simulink model "torpedo_tom_ole__09_12_19_modell"  (R2019a)
settings: Solver=ode1  StartTime=0.0  StopTime=30  FixedStep=1e-4  RelTol=1e-3
values from neighbouring files (symbols this model uses):
  K_MESS = 1.0    (= 1)    [Hausaufgabe_Schiffeversenken_zum_16_12_19_Teil1.m]    (also in Hausaufgabe_Schiffeversenken_zum_16_12_19_Teil2.m; torpedo_tom_ole__09_12_19.m; torpedo_tom_ole__25_11_19.m)
  K_r = place(ss_A_Strecke,ss_B_Strecke,Placed_Poles)    [Hausaufgabe_Schiffeversenken_zum_16_12_19_Teil2.m]    (also in torpedo_tom_ole__09_12_19.m = place(ss_A,ss_B,Placed_Poles))
  P_VORFILTER = -(ss_C_Strecke*((ss_A_Strecke-ss_B_Strecke*K_r)^-1)*ss_B_Strecke)^-1    [Hausaufgabe_Schiffeversenken_zum_16_12_19_Teil2.m]    (also in torpedo_tom_ole__09_12_19.m = -(ss_C*((ss_A-ss_B*K_r)^-1)*ss_B)^-1)
  ss_A = [0 1 0 0; 0 0 a23 0; 0 0 0 1; 0 0 a43 0]    [V2_A4_ZR_separ_nonlin_Aufgabenstellung.m]    (also in rocket_task_definition.m; torpedo_tom_ole__09_12_19.m = [-1/T_RM 0 0; K_IS/T_NOMOTO -1/T_NOMOTO 0; 0 1 0])
  ss_B = [0; b2; 0; b4]    [V2_A4_ZR_separ_nonlin_Aufgabenstellung.m]    (also in rocket_task_definition.m; torpedo_tom_ole__09_12_19.m = [K_RM/T_RM; 0; 0])
  ss_C = [1 0 0 0; 0 1 0 0; 0 0 1 0; 0 0 0 1]    [V2_A4_ZR_separ_nonlin_Aufgabenstellung.m]    (also in rocket_task_definition.m; torpedo_tom_ole__09_12_19.m = [0 0 1])
  ss_D = zeros(n,1)    [V2_A4_ZR_separ_nonlin_Aufgabenstellung.m]    (also in rocket_task_definition.m; torpedo_tom_ole__09_12_19.m = 0)
  T_MESS = 0.5    [Hausaufgabe_Schiffeversenken_zum_16_12_19_Teil1.m]    (also in Hausaufgabe_Schiffeversenken_zum_16_12_19_Teil2.m; torpedo_tom_ole__09_12_19.m; torpedo_tom_ole__25_11_19.m)
libraries: simulink x2
settings Model: Creator=setohein  LastModifiedBy=thein
settings DataIOCC: ReturnWorkspaceOutputs=off
settings DebuggingCC: ArithmeticOperatorsInVariantConditions=warning

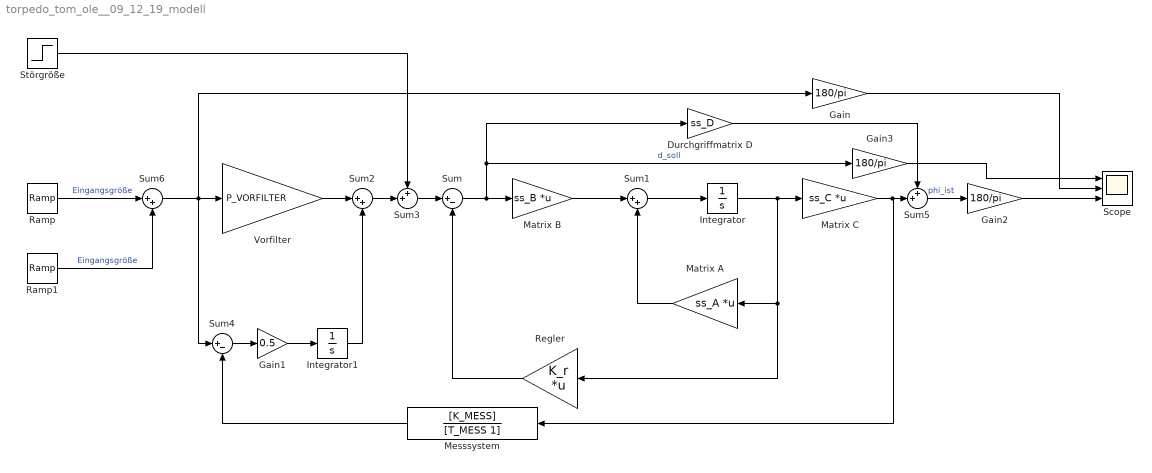
== system torpedo_tom_ole__09_12_19_modell ==
  Durchgriffmatrix D : Gain  Gain=ss_D
  Gain : Gain  Gain=180/pi
  Gain1 : Gain  Gain=0.5
  Gain2 : Gain  Gain=180/pi
  Gain3 : Gain  Gain=180/pi
  Integrator : Integrator
  Integrator1 : Integrator
  Matrix A : Gain  Gain=ss_A  Multiplication=Matrix(K*u) (u vector)
  Matrix B : Gain  Gain=ss_B  Multiplication=Matrix(K*u)
  Matrix C : Gain  Gain=ss_C  Multiplication=Matrix(K*u) (u vector)
  Messsystem : TransferFcn  Numerator=[K_MESS]  Denominator=[T_MESS 1]
  Ramp : simulink/Sources/Ramp  slope=(90*pi/180)/4  start=0  InitialOutput=0
  Ramp1 : simulink/Sources/Ramp  slope=-(90*pi/180)/4  start=4  InitialOutput=0
  Regler : Gain  Gain=K_r  Multiplication=Matrix(K*u) (u vector)
  Scope : Scope  NumInputPorts=3
  Störgröße : Step  Time=10  After=-1  SampleTime=0
  Sum : Sum  Inputs=|+-
  Sum1 : Sum  Inputs=|++
  Sum2 : Sum  Inputs=|++
  Sum3 : Sum  Inputs=++|
  Sum4 : Sum  Inputs=|+-
  Sum5 : Sum  Inputs=++|
  Sum6 : Sum  Inputs=|++
  Vorfilter : Gain  Gain=P_VORFILTER
  wires:
  Sum1/1 -> Integrator/1
  Matrix B/1 -> Sum1/1
  Integrator/1 -> Regler/1, Matrix A/1, Matrix C/1
  Matrix A/1 -> Sum1/2
  Matrix C/1 -> Messsystem/1, Sum5/2
  Sum/1 -> Durchgriffmatrix D/1, Gain3/1, Matrix B/1  "d_soll"
  Regler/1 -> Sum/2
  Ramp/1 -> Sum6/1  "Eingangsgröße"
  Sum3/1 -> Sum/1
  Vorfilter/1 -> Sum2/1
  Sum4/1 -> Gain1/1
  Gain1/1 -> Integrator1/1
  Sum5/1 -> Gain2/1  "phi_ist"
  Durchgriffmatrix D/1 -> Sum5/1
  Sum6/1 -> Vorfilter/1, Sum4/1, Gain/1
  Ramp1/1 -> Sum6/2  "Eingangsgröße"
  Gain/1 -> Scope/2
  Gain2/1 -> Scope/3
  Gain3/1 -> Scope/1
  Messsystem/1 -> Sum4/2
  Integrator1/1 -> Sum2/2
  Störgröße/1 -> Sum3/1
  Sum2/1 -> Sum3/2
